simulink subsystem "Day4_5_Scenario_1"  (R2024a)
settings: Solver=VariableStepAuto  StartTime=0.0  StopTime=10.0  RelTol=1e-3
libraries: CarMaker4SL x44
(part 1 of 5)
settings Model: Creator=junhyung.cha  LastModifiedBy=User

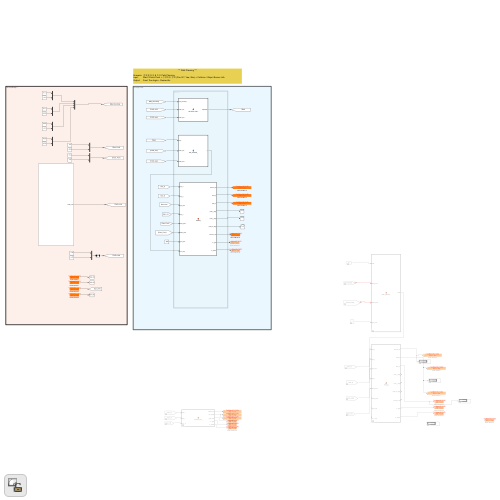
[thumbnail: Simulink's stored preview of the top-level diagram]
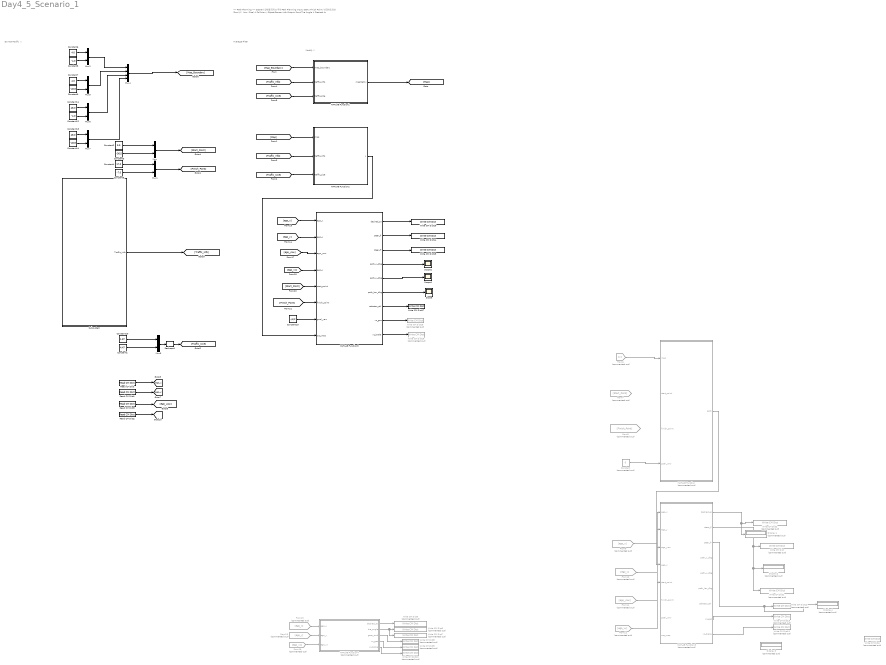
== system Day4_5_Scenario_1 ==
  note: Average Filter
  note: Do Not Modify !!
  note: Modify !!
  note: *** Path Planning ***
      |
      | Scenario: 장애물 회피 & 주차 Path Planning
      | Input: Start / Finish Point + 선행차량 정보 (Pos X/Y, Yaw, Size) + Collision / Object Sensor Info
      | Output: Front Tire Angle + Desired Ax
  Constant : Constant  Commented=on  Value=0
  Constant1 : Constant  Value=4.47
  Constant10 : Constant  Value=1.97
  Constant11 : Constant  Value=48.0
  Constant12 : Constant  Value=-4.0
  Constant13 : Constant  Value=48.0
  Constant14 : Constant  Value=-46.8
  Constant15 : Constant  Value=-pi/2
  Constant2 : Constant  Value=5.5
  Constant3 : Constant  Value=-36.5
  Constant4 : Constant  Value=17.0
  Constant5 : Constant  Value=-7.0
  Constant6 : Constant  Value=4.0
  Constant7 : Constant  Value=4.0
  Constant8 : Constant  Value=-4.0
  Constant9 : Constant  Value=-46.8
  Display{1..4} (4 alike) : Display  Commented=on
  From10 : From  Commented=on  GotoTag=ego_y
  From11 : From  Commented=on  GotoTag=ego_yaw
  From12 : From  Commented=on  GotoTag=ego_vx
  From13 : From  Commented=on  GotoTag=ego_y
  From15 : From  Commented=on  GotoTag=ego_x
  From16 : From  Commented=on  GotoTag=ego_vx
  From6 : From  Commented=on  GotoTag=y
  From7 : From  Commented=on  GotoTag=Start_Point
  From8 : From  Commented=on  GotoTag=Finish_Point
  From9 : From  Commented=on  GotoTag=ego_x
  MATLAB Function : MATLAB Function  Commented=on  TreatAsAtomicUnit=on
  MATLAB Function1 : MATLAB Function  TreatAsAtomicUnit=on
  MATLAB Function2 : MATLAB Function  TreatAsAtomicUnit=on
  MATLAB Function3 : MATLAB Function  Commented=on  TreatAsAtomicUnit=on
  MATLAB Function4 : MATLAB Function  Commented=on  TreatAsAtomicUnit=on
  MATLAB Function5 : MATLAB Function  TreatAsAtomicUnit=on
  Mux{,1..3,5..7} (7 alike) : Mux  Inputs=2
  Mux4 : Mux
  Read CM Dict : CarMaker4SL/Read CM Dict  xname=Car.Fr1.tx  xsync=off  xstime=Continuous
  Read CM Dict1 : CarMaker4SL/Read CM Dict  xname=Car.Fr1.ty  xsync=off  xstime=Continuous
  Read CM Dict2 : CarMaker4SL/Read CM Dict  xname=Car.v  xsync=off  xstime=Continuous
  Read CM Dict3 : CarMaker4SL/Read CM Dict  xname=Car.Fr1.rz  xsync=off  xstime=Continuous
  Reshape1 : Reshape  OutputDimensionality=Row vector (2-D)  OutputDimensions=[2,2]
  Scope : Scope
  Scope1 : Scope
  Scope2 : Scope
  Subsystem : Subsystem
  Write CM Dict : CarMaker4SL/Write CM Dict  Commented=on  xname=Car.CFL.rz_ext  xsync=off
  Write CM Dict1 : CarMaker4SL/Write CM Dict  Commented=on  xname=Car.CFR.rz_ext  xsync=off
  Write CM Dict10 : CarMaker4SL/Write CM Dict  Commented=on  xname=VC.Brake  xsync=off
  Write CM Dict11 : CarMaker4SL/Write CM Dict  Commented=on  xname=VC.Brake  xsync=off
  Write CM Dict12 : CarMaker4SL/Write CM Dict  Commented=on  xname=VC.SelectorCtrl  xsync=off
  Write CM Dict13 : CarMaker4SL/Write CM Dict  Commented=on  xname=VC.Gas  xsync=off
  Write CM Dict14 : CarMaker4SL/Write CM Dict  xname=Car.CFL.rz_ext  xsync=off
  Write CM Dict15 : CarMaker4SL/Write CM Dict  xname=Car.CFR.rz_ext  xsync=off
  Write CM Dict16 : CarMaker4SL/Write CM Dict  Commented=on  xname=VC.Brake  xsync=off
  Write CM Dict17 : CarMaker4SL/Write CM Dict  xname=DM.SelectorCtrl  xsync=off
  Write CM Dict18 : CarMaker4SL/Write CM Dict  Commented=on  xname=VC.Gas  xsync=off
  Write CM Dict19 : CarMaker4SL/Write CM Dict  xname=AccelCtrl.DesiredAx  xsync=off
  Write CM Dict2 : CarMaker4SL/Write CM Dict  Commented=on  xname=AccelCtrl.DesiredAx  xsync=off
  Write CM Dict4 : CarMaker4SL/Write CM Dict  Commented=on  xname=DM.SelectorCtrl  xsync=off
  Write CM Dict5 : CarMaker4SL/Write CM Dict  Commented=on  xname=AccelCtrl.DesiredAx  xsync=off
  Write CM Dict6 : CarMaker4SL/Write CM Dict  Commented=on  xname=Car.CFL.rz_ext  xsync=off
  Write CM Dict7 : CarMaker4SL/Write CM Dict  Commented=on  xname=Car.CFR.rz_ext  xsync=off
  Write CM Dict8 : CarMaker4SL/Write CM Dict  Commented=on  xname=VC.SelectorCtrl  xsync=off
  Write CM Dict9 : CarMaker4SL/Write CM Dict  Commented=on  xname=VC.Gas  xsync=off
  wires:
  [Map] -> MATLAB Function2/1(map)
  Mux/1 -> [Start_Point]
  Constant2/1 -> Mux/1
  Constant3/1 -> Mux/2
  Constant5/1 -> Mux1/2
  Mux1/1 -> [Finish_Point]
  Constant4/1 -> Mux1/1
  Constant6/1 -> Mux2/1
  Constant8/1 -> Mux2/2
  Constant9/1 -> Mux5/2
  [Map_Boundary] -> MATLAB Function1/1(map_boundary)
  Subsystem/1(Traffic_Info) -> [Traffic_Info]
  [Traffic_Info] -> MATLAB Function2/2(traffic_info)
  Mux3/1 -> Reshape1/1
  [Traffic_size] -> MATLAB Function2/3(traffic_size)
  Constant10/1 -> Mux3/1
  Constant1/1 -> Mux3/2
  Mux2/1 -> Mux4/1
  Mux5/1 -> Mux4/2
  Mux4/1 -> [Map_Boundary]
  Constant7/1 -> Mux5/1
  [Traffic_Info] -> MATLAB Function1/2(traffic_info)
  [Traffic_size] -> MATLAB Function1/3(traffic_size)
  Reshape1/1 -> [Traffic_size]
  MATLAB Function1/1(mapMatrix) -> [Map]
  MATLAB Function2/1(y) -> MATLAB Function5/8(occ_map)
  Constant11/1 -> Mux6/1
  Mux6/1 -> Mux4/3
  Constant12/1 -> Mux6/2
  Constant14/1 -> Mux7/2
  Mux7/1 -> Mux4/4
  Constant13/1 -> Mux7/1
  ? -> MATLAB Function/3(finish_point)
  ? -> MATLAB Function/2(start_point)
  From6/1 -> MATLAB Function/1(map)
  MATLAB Function3/2(steer_fl) -> Write CM Dict/1, Display2/1, Write CM Dict1/1
  Read CM Dict/1 -> [ego_x]
  Read CM Dict1/1 -> [ego_y]
  Read CM Dict3/1 -> [ego_yaw]
  Read CM Dict2/1 -> [ego_vx]
  MATLAB Function3/1(desired_ax) -> Write CM Dict2/1, Display1/1
  MATLAB Function/1(path) -> MATLAB Function3/4(ego_v)
  MATLAB Function3/3(steer_fr) -> Write CM Dict12/1, Display4/1
  From9/1 -> MATLAB Function3/1(ego_x)
  Constant/1 -> MATLAB Function/4(goal_yaw)
  From11/1 -> MATLAB Function3/3(ego_yaw)
  From10/1 -> MATLAB Function3/2(ego_y)
  From15/1 -> MATLAB Function4/1(ego_x)
  From13/1 -> MATLAB Function4/2(ego_y)
  From16/1 -> MATLAB Function4/3(ego_vx)
  MATLAB Function4/1(desired_ax) -> Write CM Dict5/1
  MATLAB Function4/2(tire_angle) -> Write CM Dict6/1, Write CM Dict7/1
  MATLAB Function4/3(gear_cmd) -> Write CM Dict8/1
  MATLAB Function4/4(vc_gas) -> Write CM Dict9/1
  MATLAB Function4/5(vc_brake) -> Write CM Dict10/1
  MATLAB Function3/8(vc_gas) -> Write CM Dict13/1
  MATLAB Function3/9(vc_brake) -> Write CM Dict11/1
  From12/1 -> MATLAB Function3/5(start_point)
  [ego_x] -> MATLAB Function5/1(ego_x)
  [ego_y] -> MATLAB Function5/2(ego_y)
  [ego_yaw] -> MATLAB Function5/3(ego_yaw)
  [ego_vx] -> MATLAB Function5/4(ego_v)
  [Finish_Point] -> MATLAB Function5/6(finish_point)
  [Start_Point] -> MATLAB Function5/5(start_point)
  Constant15/1 -> MATLAB Function5/7(goal_yaw)
  MATLAB Function5/1(desired_ax) -> Write CM Dict19/1
  MATLAB Function5/2(steer_fl) -> Write CM Dict14/1
  MATLAB Function5/3(steer_fr) -> Write CM Dict15/1
  MATLAB Function5/7(selector_ctrl) -> Write CM Dict17/1
  MATLAB Function5/8(vc_gas) -> Write CM Dict18/1
  MATLAB Function5/9(vc_brake) -> Write CM Dict16/1
  MATLAB Function5/6(path_len_dbg) -> Scope/1
  MATLAB Function5/5(path_y_dbg) -> Scope1/1
  MATLAB Function5/4(path_x_dbg) -> Scope2/1

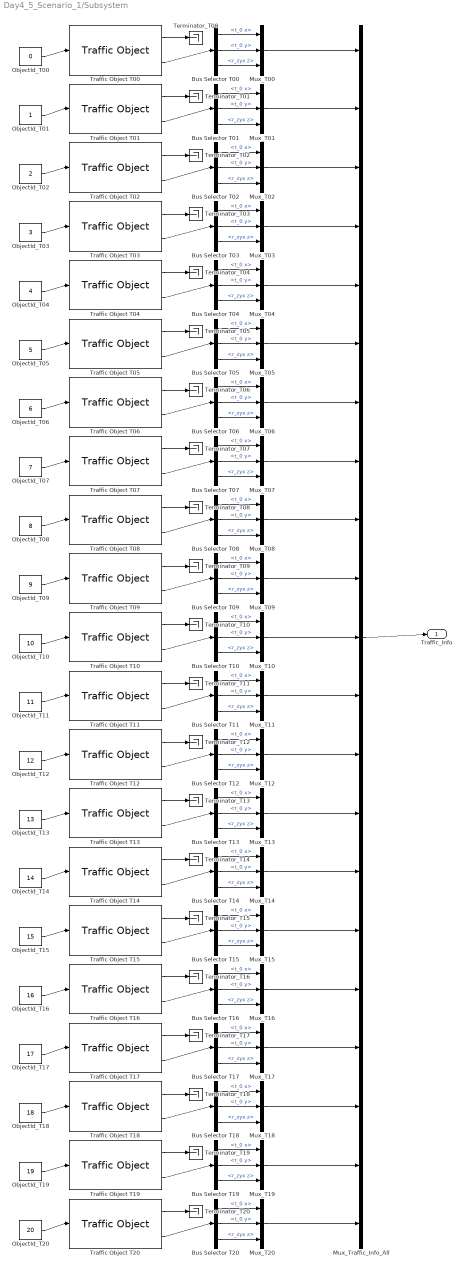
== system Day4_5_Scenario_1/Subsystem ==
  Bus Selector T00 : BusSelector  OutputSignals=t_0 x,t_0 y,r_zyx z
  Bus Selector T01 : BusSelector  OutputSignals=t_0 x,t_0 y,r_zyx z
  Bus Selector T02 : BusSelector  OutputSignals=t_0 x,t_0 y,r_zyx z
  Bus Selector T03 : BusSelector  OutputSignals=t_0 x,t_0 y,r_zyx z
  Bus Selector T04 : BusSelector  OutputSignals=t_0 x,t_0 y,r_zyx z
  Bus Selector T05 : BusSelector  OutputSignals=t_0 x,t_0 y,r_zyx z
  Bus Selector T06 : BusSelector  OutputSignals=t_0 x,t_0 y,r_zyx z
  Bus Selector T07 : BusSelector  OutputSignals=t_0 x,t_0 y,r_zyx z
  Bus Selector T08 : BusSelector  OutputSignals=t_0 x,t_0 y,r_zyx z
  Bus Selector T09 : BusSelector  OutputSignals=t_0 x,t_0 y,r_zyx z
  Bus Selector T{10..20} (11 alike) : BusSelector  OutputSignals=t_0 x,t_0 y,r_zyx z
  Mux_T00 : Mux  Inputs=3
  Mux_T01 : Mux  Inputs=3
  Mux_T02 : Mux  Inputs=3
  Mux_T03 : Mux  Inputs=3
  Mux_T04 : Mux  Inputs=3
  Mux_T05 : Mux  Inputs=3
  Mux_T06 : Mux  Inputs=3
  Mux_T07 : Mux  Inputs=3
  Mux_T08 : Mux  Inputs=3
  Mux_T09 : Mux  Inputs=3
  Mux_T{10..20} (11 alike) : Mux  Inputs=3
  Mux_Traffic_Info_All : Mux  Inputs=21
  ObjectId_T00 : Constant  Value=0
  ObjectId_T01 : Constant
  ObjectId_T02 : Constant  Value=2
  ObjectId_T03 : Constant  Value=3
  ObjectId_T04 : Constant  Value=4
  ObjectId_T05 : Constant  Value=5
  ObjectId_T06 : Constant  Value=6
  ObjectId_T07 : Constant  Value=7
  ObjectId_T08 : Constant  Value=8
  ObjectId_T09 : Constant  Value=9
  ObjectId_T10 : Constant  Value=10
  ObjectId_T11 : Constant  Value=11
  ObjectId_T12 : Constant  Value=12
  ObjectId_T13 : Constant  Value=13
  ObjectId_T14 : Constant  Value=14
  ObjectId_T15 : Constant  Value=15
  ObjectId_T16 : Constant  Value=16
  ObjectId_T17 : Constant  Value=17
  ObjectId_T18 : Constant  Value=18
  ObjectId_T19 : Constant  Value=19
  ObjectId_T20 : Constant  Value=20
  Terminator_T00 : Terminator
  Terminator_T01 : Terminator
  Terminator_T02 : Terminator
  Terminator_T03 : Terminator
  Terminator_T04 : Terminator
  Terminator_T05 : Terminator
  Terminator_T06 : Terminator
  Terminator_T07 : Terminator
  Terminator_T08 : Terminator
  Terminator_T09 : Terminator
  Terminator_T{10..20} (11 alike) : Terminator
  Traffic Object T00 : CarMaker4SL/Traffic Object  xname=T00  ximode=Traffic Id  xstime=Inherited
      settings: SourceProductName=CarMaker4SL
  Traffic Object T01 : CarMaker4SL/Traffic Object  xname=T01  ximode=Traffic Id  xstime=Inherited
      settings: SourceProductName=CarMaker4SL
  Traffic Object T02 : CarMaker4SL/Traffic Object  xname=T02  ximode=Traffic Id  xstime=Inherited
      settings: SourceProductName=CarMaker4SL
  Traffic Object T03 : CarMaker4SL/Traffic Object  xname=T03  ximode=Traffic Id  xstime=Inherited
      settings: SourceProductName=CarMaker4SL
  Traffic Object T04 : CarMaker4SL/Traffic Object  xname=T04  ximode=Traffic Id  xstime=Inherited
      settings: SourceProductName=CarMaker4SL
  Traffic Object T05 : CarMaker4SL/Traffic Object  xname=T05  ximode=Traffic Id  xstime=Inherited
      settings: SourceProductName=CarMaker4SL
  Traffic Object T06 : CarMaker4SL/Traffic Object  xname=T06  ximode=Traffic Id  xstime=Inherited
      settings: SourceProductName=CarMaker4SL
  Traffic Object T07 : CarMaker4SL/Traffic Object  xname=T07  ximode=Traffic Id  xstime=Inherited
      settings: SourceProductName=CarMaker4SL
  Traffic Object T08 : CarMaker4SL/Traffic Object  xname=T08  ximode=Traffic Id  xstime=Inherited
      settings: SourceProductName=CarMaker4SL
  Traffic Object T09 : CarMaker4SL/Traffic Object  xname=T09  ximode=Traffic Id  xstime=Inherited
      settings: SourceProductName=CarMaker4SL
  Traffic Object T10 : CarMaker4SL/Traffic Object  xname=T10  ximode=Traffic Id  xstime=Inherited
      settings: SourceProductName=CarMaker4SL
  Traffic Object T11 : CarMaker4SL/Traffic Object  xname=T11  ximode=Traffic Id  xstime=Inherited
      settings: SourceProductName=CarMaker4SL
  Traffic Object T12 : CarMaker4SL/Traffic Object  xname=T12  ximode=Traffic Id  xstime=Inherited
      settings: SourceProductName=CarMaker4SL
  Traffic Object T13 : CarMaker4SL/Traffic Object  xname=T13  ximode=Traffic Id  xstime=Inherited
      settings: SourceProductName=CarMaker4SL
  Traffic Object T14 : CarMaker4SL/Traffic Object  xname=T14  ximode=Traffic Id  xstime=Inherited
      settings: SourceProductName=CarMaker4SL
  Traffic Object T15 : CarMaker4SL/Traffic Object  xname=T15  ximode=Traffic Id  xstime=Inherited
      settings: SourceProductName=CarMaker4SL
  Traffic Object T16 : CarMaker4SL/Traffic Object  xname=T16  ximode=Traffic Id  xstime=Inherited
      settings: SourceProductName=CarMaker4SL
  Traffic Object T17 : CarMaker4SL/Traffic Object  xname=T17  ximode=Traffic Id  xstime=Inherited
      settings: SourceProductName=CarMaker4SL
  Traffic Object T18 : CarMaker4SL/Traffic Object  xname=T18  ximode=Traffic Id  xstime=Inherited
      settings: SourceProductName=CarMaker4SL
  Traffic Object T19 : CarMaker4SL/Traffic Object  xname=T19  ximode=Traffic Id  xstime=Inherited
      settings: SourceProductName=CarMaker4SL
  Traffic Object T20 : CarMaker4SL/Traffic Object  xname=T20  ximode=Traffic Id  xstime=Inherited
      settings: SourceProductName=CarMaker4SL
  Traffic_Info : Outport
  wires:
  ObjectId_T00/1 -> Traffic Object T00/1
  Traffic Object T00/1 -> Terminator_T00/1
  Traffic Object T00/2 -> Bus Selector T00/1
  Bus Selector T00/1 -> Mux_T00/1  "<t_0 x>"
  Bus Selector T00/2 -> Mux_T00/2  "<t_0 y>"
  Bus Selector T00/3 -> Mux_T00/3  "<r_zyx z>"
  ObjectId_T01/1 -> Traffic Object T01/1
  Traffic Object T01/1 -> Terminator_T01/1
  Traffic Object T01/2 -> Bus Selector T01/1
  Bus Selector T01/1 -> Mux_T01/1  "<t_0 x>"
  Bus Selector T01/2 -> Mux_T01/2  "<t_0 y>"
  Bus Selector T01/3 -> Mux_T01/3  "<r_zyx z>"
  ObjectId_T02/1 -> Traffic Object T02/1
  Traffic Object T02/1 -> Terminator_T02/1
  Traffic Object T02/2 -> Bus Selector T02/1
  Bus Selector T02/1 -> Mux_T02/1  "<t_0 x>"
  Bus Selector T02/2 -> Mux_T02/2  "<t_0 y>"
  Bus Selector T02/3 -> Mux_T02/3  "<r_zyx z>"
  ObjectId_T03/1 -> Traffic Object T03/1
  Traffic Object T03/1 -> Terminator_T03/1
  Traffic Object T03/2 -> Bus Selector T03/1
  Bus Selector T03/1 -> Mux_T03/1  "<t_0 x>"
  Bus Selector T03/2 -> Mux_T03/2  "<t_0 y>"
  Bus Selector T03/3 -> Mux_T03/3  "<r_zyx z>"
  ObjectId_T04/1 -> Traffic Object T04/1
  Traffic Object T04/1 -> Terminator_T04/1
  Traffic Object T04/2 -> Bus Selector T04/1
  Bus Selector T04/1 -> Mux_T04/1  "<t_0 x>"
  Bus Selector T04/2 -> Mux_T04/2  "<t_0 y>"
  Bus Selector T04/3 -> Mux_T04/3  "<r_zyx z>"
  ObjectId_T05/1 -> Traffic Object T05/1
  Traffic Object T05/1 -> Terminator_T05/1
  Traffic Object T05/2 -> Bus Selector T05/1
  Bus Selector T05/1 -> Mux_T05/1  "<t_0 x>"
  Bus Selector T05/2 -> Mux_T05/2  "<t_0 y>"
  Bus Selector T05/3 -> Mux_T05/3  "<r_zyx z>"
  ObjectId_T06/1 -> Traffic Object T06/1
  Traffic Object T06/1 -> Terminator_T06/1
  Traffic Object T06/2 -> Bus Selector T06/1
  Bus Selector T06/1 -> Mux_T06/1  "<t_0 x>"
  Bus Selector T06/2 -> Mux_T06/2  "<t_0 y>"
  Bus Selector T06/3 -> Mux_T06/3  "<r_zyx z>"
  ObjectId_T07/1 -> Traffic Object T07/1
  Traffic Object T07/1 -> Terminator_T07/1
  Traffic Object T07/2 -> Bus Selector T07/1
  Bus Selector T07/1 -> Mux_T07/1  "<t_0 x>"
  Bus Selector T07/2 -> Mux_T07/2  "<t_0 y>"
  Bus Selector T07/3 -> Mux_T07/3  "<r_zyx z>"
  ObjectId_T08/1 -> Traffic Object T08/1
  Traffic Object T08/1 -> Terminator_T08/1
  Traffic Object T08/2 -> Bus Selector T08/1
  Bus Selector T08/1 -> Mux_T08/1  "<t_0 x>"
  Bus Selector T08/2 -> Mux_T08/2  "<t_0 y>"
  Bus Selector T08/3 -> Mux_T08/3  "<r_zyx z>"
  ObjectId_T09/1 -> Traffic Object T09/1
  Traffic Object T09/1 -> Terminator_T09/1
  Traffic Object T09/2 -> Bus Selector T09/1
  Bus Selector T09/1 -> Mux_T09/1  "<t_0 x>"
  Bus Selector T09/2 -> Mux_T09/2  "<t_0 y>"
  Bus Selector T09/3 -> Mux_T09/3  "<r_zyx z>"
  ObjectId_T10/1 -> Traffic Object T10/1
  Traffic Object T10/1 -> Terminator_T10/1
  Traffic Object T10/2 -> Bus Selector T10/1
  Bus Selector T10/1 -> Mux_T10/1  "<t_0 x>"
  Bus Selector T10/2 -> Mux_T10/2  "<t_0 y>"
  Bus Selector T10/3 -> Mux_T10/3  "<r_zyx z>"
  ObjectId_T11/1 -> Traffic Object T11/1
  Traffic Object T11/1 -> Terminator_T11/1
  Traffic Object T11/2 -> Bus Selector T11/1
  Bus Selector T11/1 -> Mux_T11/1  "<t_0 x>"
  Bus Selector T11/2 -> Mux_T11/2  "<t_0 y>"
  Bus Selector T11/3 -> Mux_T11/3  "<r_zyx z>"
  ObjectId_T12/1 -> Traffic Object T12/1
  Traffic Object T12/1 -> Terminator_T12/1
  Traffic Object T12/2 -> Bus Selector T12/1
  Bus Selector T12/1 -> Mux_T12/1  "<t_0 x>"
  Bus Selector T12/2 -> Mux_T12/2  "<t_0 y>"
  Bus Selector T12/3 -> Mux_T12/3  "<r_zyx z>"
  ObjectId_T13/1 -> Traffic Object T13/1
  Traffic Object T13/1 -> Terminator_T13/1
  Traffic Object T13/2 -> Bus Selector T13/1
  Bus Selector T13/1 -> Mux_T13/1  "<t_0 x>"
  Bus Selector T13/2 -> Mux_T13/2  "<t_0 y>"
  Bus Selector T13/3 -> Mux_T13/3  "<r_zyx z>"
  ObjectId_T14/1 -> Traffic Object T14/1
  Traffic Object T14/1 -> Terminator_T14/1
  Traffic Object T14/2 -> Bus Selector T14/1
  Bus Selector T14/1 -> Mux_T14/1  "<t_0 x>"
  Bus Selector T14/2 -> Mux_T14/2  "<t_0 y>"
  Bus Selector T14/3 -> Mux_T14/3  "<r_zyx z>"
  ObjectId_T15/1 -> Traffic Object T15/1
  Traffic Object T15/1 -> Terminator_T15/1
  Traffic Object T15/2 -> Bus Selector T15/1
  Bus Selector T15/1 -> Mux_T15/1  "<t_0 x>"
  Bus Selector T15/2 -> Mux_T15/2  "<t_0 y>"
  Bus Selector T15/3 -> Mux_T15/3  "<r_zyx z>"
  ObjectId_T16/1 -> Traffic Object T16/1
  Traffic Object T16/1 -> Terminator_T16/1
  Traffic Object T16/2 -> Bus Selector T16/1
  Bus Selector T16/1 -> Mux_T16/1  "<t_0 x>"
  Bus Selector T16/2 -> Mux_T16/2  "<t_0 y>"
  Bus Selector T16/3 -> Mux_T16/3  "<r_zyx z>"
  ObjectId_T17/1 -> Traffic Object T17/1
  Traffic Object T17/1 -> Terminator_T17/1
  Traffic Object T17/2 -> Bus Selector T17/1
  Bus Selector T17/1 -> Mux_T17/1  "<t_0 x>"
  Bus Selector T17/2 -> Mux_T17/2  "<t_0 y>"
  Bus Selector T17/3 -> Mux_T17/3  "<r_zyx z>"
  ObjectId_T18/1 -> Traffic Object T18/1
  Traffic Object T18/1 -> Terminator_T18/1
  Traffic Object T18/2 -> Bus Selector T18/1
  Bus Selector T18/1 -> Mux_T18/1  "<t_0 x>"
  Bus Selector T18/2 -> Mux_T18/2  "<t_0 y>"
  Bus Selector T18/3 -> Mux_T18/3  "<r_zyx z>"
  ObjectId_T19/1 -> Traffic Object T19/1
  Traffic Object T19/1 -> Terminator_T19/1
  Traffic Object T19/2 -> Bus Selector T19/1
  Bus Selector T19/1 -> Mux_T19/1  "<t_0 x>"
  Bus Selector T19/2 -> Mux_T19/2  "<t_0 y>"
  Bus Selector T19/3 -> Mux_T19/3  "<r_zyx z>"
  ObjectId_T20/1 -> Traffic Object T20/1
  Traffic Object T20/1 -> Terminator_T20/1
  Traffic Object T20/2 -> Bus Selector T20/1
  Bus Selector T20/1 -> Mux_T20/1  "<t_0 x>"
  Bus Selector T20/2 -> Mux_T20/2  "<t_0 y>"
  Bus Selector T20/3 -> Mux_T20/3  "<r_zyx z>"
  Mux_T00/1 -> Mux_Traffic_Info_All/1
  Mux_T01/1 -> Mux_Traffic_Info_All/2
  Mux_T02/1 -> Mux_Traffic_Info_All/3
  Mux_T03/1 -> Mux_Traffic_Info_All/4
  Mux_T04/1 -> Mux_Traffic_Info_All/5
  Mux_T05/1 -> Mux_Traffic_Info_All/6
  Mux_T06/1 -> Mux_Traffic_Info_All/7
  Mux_T07/1 -> Mux_Traffic_Info_All/8
  Mux_T08/1 -> Mux_Traffic_Info_All/9
  Mux_T09/1 -> Mux_Traffic_Info_All/10
  Mux_T10/1 -> Mux_Traffic_Info_All/11
  Mux_T11/1 -> Mux_Traffic_Info_All/12
  Mux_T12/1 -> Mux_Traffic_Info_All/13
  Mux_T13/1 -> Mux_Traffic_Info_All/14
  Mux_T14/1 -> Mux_Traffic_Info_All/15
  Mux_T15/1 -> Mux_Traffic_Info_All/16
  Mux_T16/1 -> Mux_Traffic_Info_All/17
  Mux_T17/1 -> Mux_Traffic_Info_All/18
  Mux_T18/1 -> Mux_Traffic_Info_All/19
  Mux_T19/1 -> Mux_Traffic_Info_All/20
  Mux_T20/1 -> Mux_Traffic_Info_All/21
  Mux_Traffic_Info_All/1 -> Traffic_Info/1
